simulink subsystem "SCDynamics"  (R2021a)
settings: Solver=VariableStepAuto  StartTime=0.0  StopTime=10.0  RelTol=1e-3
undefined symbols (not defined in the file): Ix, Iy, Iz, mu, q0, r0, v0, w0
libraries: aerolibutil x2
settings Model: Creator=Laura  LastModifiedBy=Laura

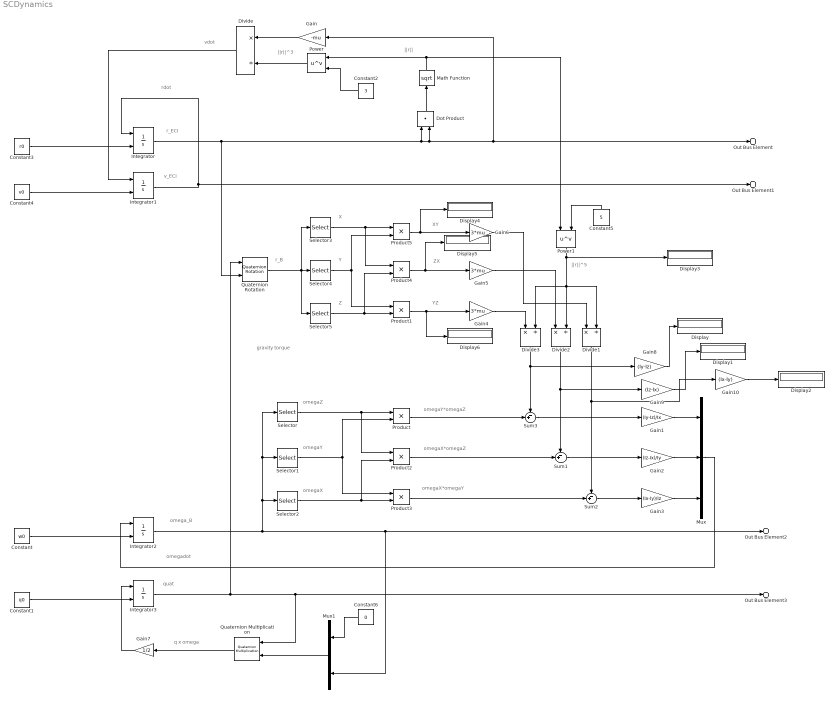
== system SCDynamics ==
  note: omegaX*omegaZ
  note: q x omega
  note: omegaX*omegaY
  note: omegaZ
  note: quat
  note: Y
  note: r_B
  note: v_ECI
  note: ZX
  note: X
  note: ||r||^3
  note: gravity torque
  note: Z
  note: omegaY*omegaZ
  note: omegaY
  note: omega_B
  note: YZ
  note: ||r||
  note: omegadot
  note: omegaX
  note: vdot
  note: r_ECI
  note: ||r||^5
  note: rdot
  note: XY
  Constant : Constant  Value=w0
  Constant1 : Constant  Value=q0
  Constant2 : Constant  Value=3
  Constant3 : Constant  Value=r0
  Constant4 : Constant  Value=v0
  Constant5 : Constant  Value=5
  Constant6 : Constant  Value=0
  Display{,1..6} (7 alike) : Display
  Divide{,1..3} (4 alike) : Product  Inputs=*/
  Dot Product : DotProduct  InputSameDT=on  OutDataTypeStr=Inherit: Inherit via internal rule
  Gain : Gain  Gain=-mu
  Gain1 : Gain  Gain=(Iy-Iz)/Ix
  Gain10 : Gain  Gain=(Ix-Iy)
  Gain2 : Gain  Gain=(Iz-Ix)/Iy
  Gain3 : Gain  Gain=(Ix-Iy)/Iz
  Gain4 : Gain  Gain=3*mu
  Gain5 : Gain  Gain=3*mu
  Gain6 : Gain  Gain=3*mu
  Gain7 : Gain  Gain=1/2
  Gain8 : Gain  Gain=(Iy-Iz)
  Gain9 : Gain  Gain=(Iz-Ix)
  Integrator{,1..3} (4 alike) : Integrator  InitialConditionSource=external
  Math Function : Math  Operator=sqrt  SignedPower=on  SaturateOnIntegerOverflow=on
  Mux : Mux  Inputs=3
  Mux1 : Mux  Inputs=2
  Power : Math  Operator=pow  SaturateOnIntegerOverflow=on
  Power1 : Math  Operator=pow  SaturateOnIntegerOverflow=on
  Product{,1..5} (6 alike) : Product
  Quaternion Multiplication : aerolibutil/Quaternion Multiplication
  Quaternion Rotation : aerolibutil/Quaternion Rotation
  Selector : Selector  InputPortWidth=3  IndexOptions=Index vector (dialog)  Indices=[3]  OutputSizes=1
  Selector1 : Selector  InputPortWidth=3  IndexOptions=Index vector (dialog)  Indices=[2]  OutputSizes=1
  Selector2 : Selector  InputPortWidth=3  IndexOptions=Index vector (dialog)  Indices=[1]  OutputSizes=1
  Selector3 : Selector  InputPortWidth=3  IndexOptions=Index vector (dialog)  Indices=[1]  OutputSizes=1
  Selector4 : Selector  InputPortWidth=3  IndexOptions=Index vector (dialog)  Indices=[2]  OutputSizes=1
  Selector5 : Selector  InputPortWidth=3  IndexOptions=Index vector (dialog)  Indices=[3]  OutputSizes=1
  Sum1 : Sum  Inputs=-+|
  Sum2 : Sum  Inputs=-+|
  Sum3 : Sum  Inputs=-+|
  Out Bus Element : Outport  PortName=DynamicsOut  Element=r_ECI
  Out Bus Element1 : Outport  PortName=DynamicsOut  Element=v_ECI
  Out Bus Element2 : Outport  PortName=DynamicsOut  Element=omega_B
  Out Bus Element3 : Outport  PortName=DynamicsOut  Element=quat
  wires:
  Selector5/1 -> Product1/2, Product4/2
  Constant1/1 -> Integrator3/2
  Gain3/1 -> Mux/3
  Power/1 -> Divide/2
  Selector2/1 -> Product3/2, Product2/2
  Integrator2/1 -> Out Bus Element2/1, Mux1/2, Selector/1, Selector1/1, Selector2/1
  Gain4/1 -> Divide3/1
  Selector4/1 -> Product1/1, Product5/2
  Constant6/1 -> Mux1/1
  Divide2/1 -> Sum1/1, Gain9/1
  Selector3/1 -> Product4/1, Product5/1
  Integrator3/1 -> Out Bus Element3/1, Quaternion Multiplication/1, Quaternion Rotation/1
  Dot Product/1 -> Math Function/1
  Divide3/1 -> Sum3/1, Gain8/1
  Integrator1/1 -> Out Bus Element1/1, Integrator/1
  Quaternion Multiplication/1 -> Gain7/1
  Quaternion Rotation/1 -> Selector5/1, Selector3/1, Selector4/1
  Mux/1 -> Integrator2/1
  Product5/1 -> Gain6/1, Display4/1
  Constant3/1 -> Integrator/2
  Gain1/1 -> Mux/1
  Gain/1 -> Divide/1
  Integrator/1 -> Dot Product/1, Dot Product/2, Out Bus Element/1, Gain/1, Quaternion Rotation/2
  Constant5/1 -> Power1/2
  Power1/1 -> Divide1/2, Divide3/2, Divide2/2, Display3/1
  Constant4/1 -> Integrator1/2
  Sum1/1 -> Gain2/1
  Sum2/1 -> Gain3/1
  Mux1/1 -> Quaternion Multiplication/2
  Gain6/1 -> Divide1/1
  Product4/1 -> Gain5/1, Display5/1
  Selector/1 -> Product/1, Product2/1
  Gain5/1 -> Divide2/1
  Sum3/1 -> Gain1/1
  Product2/1 -> Sum1/2
  Constant/1 -> Integrator2/2
  Divide1/1 -> Gain10/1, Sum2/1
  Product/1 -> Sum3/2
  Gain7/1 -> Integrator3/1
  Divide/1 -> Integrator1/1
  Constant2/1 -> Power/2
  Product3/1 -> Sum2/2
  Selector1/1 -> Product3/1, Product/2
  Gain2/1 -> Mux/2
  Math Function/1 -> Power/1, Power1/1
  Gain8/1 -> Display/1
  Gain9/1 -> Display1/1
  Gain10/1 -> Display2/1
  Product1/1 -> Gain4/1, Display6/1
